simulink model "power_PVArray_PartialShading_Project"  (R2015a)
settings: Solver=ode23tb  SolverMode=SingleTasking  StartTime=0.0  StopTime=3  FixedStep=Ts_Power  RelTol=1e-4
PreLoadFcn:
  | Ts_Power=50e-6;
  | Slope_Vdc=1;
InitFcn:
  | Ts_Power=50e-6;
  | Tc=1e-5;%break algebraic loop time constant
  | BlockName=[gcs,'/4X4 PV Array/PV cells 1'];
  | ModuleName=get_param(BlockName,'ModuleName');
  | Voc1=str2num(get_param(BlockName,'Voc'));
  | Nser1=str2num(get_param(BlockName,'Nser'));
  | Slope_Vdc=Nser1*Voc1;
StopFcn:
  | if exist('I','var') && exist('V','var')
  |    figure(1)
  |    clf
  |    n=find(I>=0);
  |    n=n(end);
  |    Vglobal=V(1:n);
  |    Iglobal=I(1:n);
  | 
  | 
  |    Pglobal=Vglobal.*Iglobal;
  |    n=find(Pglobal==max(Pglobal));
  |    Pmax=Pglobal(n);
  |    Vmp=Vglobal(n);
  |    Imp=Iglobal(n);
  | 
  | 
  |    subplot(211)
  |    plot(Vglobal, Iglobal,Vmp,Imp,'or')
  |    ylabel('Current (A)')
  |    title(sprintf('Global I-V & P-V characteristics\n %s' ,ModuleName))
  | 
  | 
  |    subplot(212)
  |    plot(Vglobal, Pglobal,Vmp,Pmax,'or')
  |    ylabel('Power (W)')
  |    xlabel('Voltage (V)')
  | end
libraries: powerlib x20, re_lib x16, simulink x1
Description:
  | Copyright 2008-2015 The MathWorks, Inc.
settings Model: CovSFcnEnable=off  Creator=MathWorks  LastModifiedBy=Student
settings SolverCC: AlgebraicLoopSolver=LineSearch
settings DataIOCC: SignalLoggingSaveFormat=ModelDataLogs
settings OptimizationCC: ExpressionDepthLimit=2147483647
settings DebuggingCC: UnderspecifiedInitializationDetection=Classic  MergeDetectMultiDrivingBlocksExec=none  MaxConsecutiveZCsMsg=none  SolverPrmCheckMsg=warning  FcnCallInpInsideContextMsg=EnableAllAsWarning  StateNameClashWarn=warning
settings GRTTargetCC: CombineOutputUpdateFcns=off  GRTInterface=on

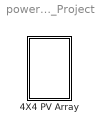
== system power_PVArray_PartialShading_Project ==
  4X4 PV Array : Subsystem  mask{Shade_A=900, Shade_B=600, Shade_C=300, Shade_D=100, No_Shade=1000}
      mask prompts: Shade_A "Shade - A"; Shade_B "Shade - B"; Shade_C "Shade - C"; Shade_D "Shade - D"

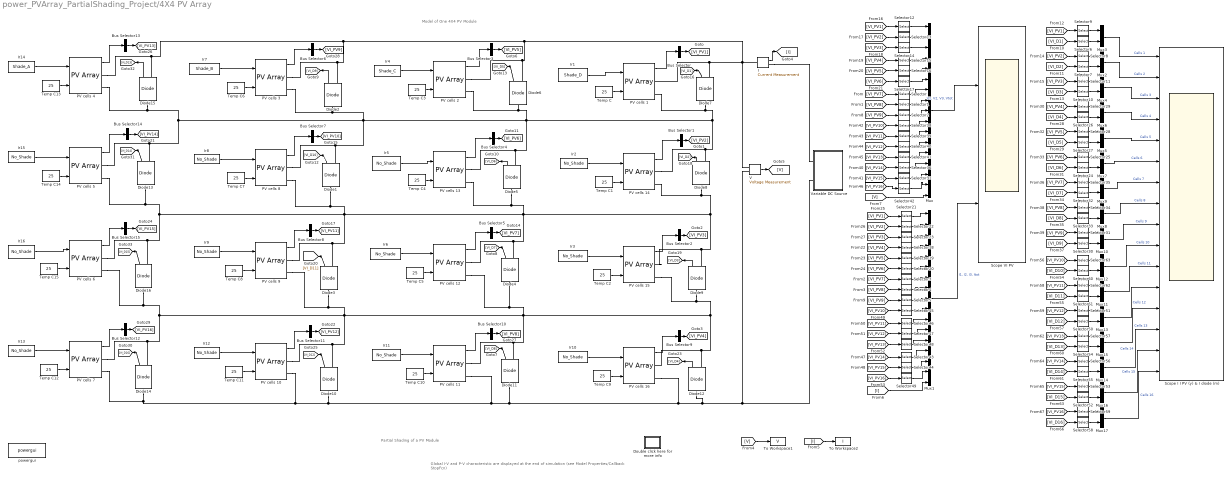
== system power_PVArray_PartialShading_Project/4X4 PV Array ==
  note: Model of One 4X4 PV Module
  note: Global I-V and P-V characteristic are displayed at the end of simulation
      | (see Model Properties/Callback StopFcn)
  note: Partial Shading of a PV Module
  Bus Selector{,1..15} (16 alike) : BusSelector  OutputSignals=V_PV,I_PV  OutputAsBus=on
  Diode{1..16} (16 alike) : powerlib/Power Electronics/Diode  Ron=0.001  Lon=0  Vf=0.7  IC=0  UseSnubber=off  Rs=1e5*inf  Cs=inf  Measurements=on
  Double click here for more info : Subsystem
      settings: OpenFcn=showdemo(bdroot(gcb))
      mask Display: disp('?')
  I : powerlib/Measurements/Current Measurement  PhasorSimulation=off  OutputType=Complex  PSBequivalent=0
  Ir1 : Constant  Value=Shade_D
  Ir{2..3,5..6,8..13,15..16} (12 alike) : Constant  Value=No_Shade
  Ir14 : Constant  Value=Shade_A
  Ir4 : Constant  Value=Shade_C
  Ir7 : Constant  Value=Shade_B
  Mux : Mux  Inputs=17
  Mux1 : Mux  Inputs=17
  Mux{2..17} (16 alike) : Mux  Inputs=2
  PV cells 1 : re_lib/Solar/PV Array  Npar=1  Nser=1  PlotType=array @ 25 deg.C & specified irradiances  S_vec="[ 1000  500  100 ]"  Temp_C_vec="[ 45 25  ]"  ModuleName=User-defined  PlotWhenSelected=off  Pm=2.2246  Ncell=1  Voc=0.7  Isc=4.74  Vm=17.64/36  Im=4.54  beta_Voc_pc=-0.33969  alpha_Isc_pc=0.063701  beta_Voc=-0.0023778  alpha_Isc=0.0030194  IL=4.8525  I0=7.8378e-11  nI=1.0965  Rsh=418.8028  Rs=0.030154  BAL=on  Tc=1  Tfilter=5e-5
      link override Diode Rsh/BAL/Transfer Fcn: Denominator="[Tc  1]"  AbsoluteTolerance=1e-3
  PV cells 10 : re_lib/Solar/PV Array  Npar=1  Nser=1  PlotType=array @ 25 deg.C & specified irradiances  S_vec="[ 1000  500  100 ]"  Temp_C_vec="[ 45 25  ]"  ModuleName=User-defined  PlotWhenSelected=off  Pm=2.2246  Ncell=1  Voc=0.7  Isc=4.74  Vm=17.64/36  Im=4.54  beta_Voc_pc=-0.33969  alpha_Isc_pc=0.063701  beta_Voc=-0.0023778  alpha_Isc=0.0030194  IL=4.8525  I0=7.8378e-11  nI=1.0965  Rsh=418.8028  Rs=0.030154  BAL=on  Tc=1  Tfilter=5e-5
      link override Diode Rsh/BAL/Transfer Fcn: Denominator="[Tc  1]"  AbsoluteTolerance=1e-3
  PV cells 11 : re_lib/Solar/PV Array  Npar=1  Nser=1  PlotType=array @ 25 deg.C & specified irradiances  S_vec="[ 1000  500  100 ]"  Temp_C_vec="[ 45 25  ]"  ModuleName=User-defined  PlotWhenSelected=off  Pm=2.2246  Ncell=1  Voc=0.7  Isc=4.74  Vm=17.64/36  Im=4.54  beta_Voc_pc=-0.33969  alpha_Isc_pc=0.063701  beta_Voc=-0.0023778  alpha_Isc=0.0030194  IL=4.8525  I0=7.8378e-11  nI=1.0965  Rsh=418.8028  Rs=0.030154  BAL=on  Tc=1  Tfilter=5e-5
      link override Diode Rsh/BAL/Transfer Fcn: Denominator="[Tc  1]"  AbsoluteTolerance=1e-3
  PV cells 12 : re_lib/Solar/PV Array  Npar=1  Nser=1  PlotType=array @ 25 deg.C & specified irradiances  S_vec="[ 1000  500  100 ]"  Temp_C_vec="[ 45 25  ]"  ModuleName=User-defined  PlotWhenSelected=off  Pm=2.2246  Ncell=1  Voc=0.7  Isc=4.74  Vm=17.64/36  Im=4.54  beta_Voc_pc=-0.33969  alpha_Isc_pc=0.063701  beta_Voc=-0.0023778  alpha_Isc=0.0030194  IL=4.8525  I0=7.8378e-11  nI=1.0965  Rsh=418.8028  Rs=0.030154  BAL=on  Tc=1  Tfilter=5e-5
      link override Diode Rsh/BAL/Transfer Fcn: Denominator="[Tc  1]"  AbsoluteTolerance=1e-3
  PV cells 13 : re_lib/Solar/PV Array  Npar=1  Nser=1  PlotType=array @ 25 deg.C & specified irradiances  S_vec="[ 1000  500  100 ]"  Temp_C_vec="[ 45 25  ]"  ModuleName=User-defined  PlotWhenSelected=off  Pm=2.2246  Ncell=1  Voc=0.7  Isc=4.74  Vm=17.64/36  Im=4.54  beta_Voc_pc=-0.33969  alpha_Isc_pc=0.063701  beta_Voc=-0.0023778  alpha_Isc=0.0030194  IL=4.8525  I0=7.8378e-11  nI=1.0965  Rsh=418.8028  Rs=0.030154  BAL=on  Tc=1  Tfilter=5e-5
      link override Diode Rsh/BAL/Transfer Fcn: Denominator="[Tc  1]"  AbsoluteTolerance=1e-3
  PV cells 14 : re_lib/Solar/PV Array  Npar=1  Nser=1  PlotType=array @ 25 deg.C & specified irradiances  S_vec="[ 1000  500  100 ]"  Temp_C_vec="[ 45 25  ]"  ModuleName=User-defined  PlotWhenSelected=off  Pm=2.2246  Ncell=1  Voc=0.7  Isc=4.74  Vm=17.64/36  Im=4.54  beta_Voc_pc=-0.33969  alpha_Isc_pc=0.063701  beta_Voc=-0.0023778  alpha_Isc=0.0030194  IL=4.8525  I0=7.8378e-11  nI=1.0965  Rsh=418.8028  Rs=0.030154  BAL=on  Tc=1  Tfilter=5e-5
      link override Diode Rsh/BAL/Transfer Fcn: Denominator="[Tc  1]"  AbsoluteTolerance=1e-3
  PV cells 15 : re_lib/Solar/PV Array  Npar=1  Nser=1  PlotType=array @ 25 deg.C & specified irradiances  S_vec="[ 1000  500  100 ]"  Temp_C_vec="[ 45 25  ]"  ModuleName=User-defined  PlotWhenSelected=off  Pm=2.2246  Ncell=1  Voc=0.7  Isc=4.74  Vm=17.64/36  Im=4.54  beta_Voc_pc=-0.33969  alpha_Isc_pc=0.063701  beta_Voc=-0.0023778  alpha_Isc=0.0030194  IL=4.8525  I0=7.8378e-11  nI=1.0965  Rsh=418.8028  Rs=0.030154  BAL=on  Tc=1  Tfilter=5e-5
      link override Diode Rsh/BAL/Transfer Fcn: Denominator="[Tc  1]"  AbsoluteTolerance=1e-3
  PV cells 16 : re_lib/Solar/PV Array  Npar=1  Nser=1  PlotType=array @ 25 deg.C & specified irradiances  S_vec="[ 1000  500  100 ]"  Temp_C_vec="[ 45 25  ]"  ModuleName=User-defined  PlotWhenSelected=off  Pm=2.2246  Ncell=1  Voc=0.7  Isc=4.74  Vm=17.64/36  Im=4.54  beta_Voc_pc=-0.33969  alpha_Isc_pc=0.063701  beta_Voc=-0.0023778  alpha_Isc=0.0030194  IL=4.8525  I0=7.8378e-11  nI=1.0965  Rsh=418.8028  Rs=0.030154  BAL=on  Tc=1  Tfilter=5e-5
      link override Diode Rsh/BAL/Transfer Fcn: Denominator="[Tc  1]"  AbsoluteTolerance=1e-3
  PV cells 2 : re_lib/Solar/PV Array  Npar=1  Nser=1  PlotType=array @ 25 deg.C & specified irradiances  S_vec="[ 1000  500  100 ]"  Temp_C_vec="[ 45 25  ]"  ModuleName=User-defined  PlotWhenSelected=off  Pm=2.2246  Ncell=1  Voc=0.7  Isc=4.74  Vm=17.64/36  Im=4.54  beta_Voc_pc=-0.33969  alpha_Isc_pc=0.063701  beta_Voc=-0.0023778  alpha_Isc=0.0030194  IL=4.8525  I0=7.8378e-11  nI=1.0965  Rsh=418.8028  Rs=0.030154  BAL=on  Tc=1  Tfilter=5e-5
      link override Diode Rsh/BAL/Transfer Fcn: Denominator="[Tc  1]"  AbsoluteTolerance=1e-3
  PV cells 3 : re_lib/Solar/PV Array  Npar=1  Nser=1  PlotType=array @ 25 deg.C & specified irradiances  S_vec="[ 1000  500  100 ]"  Temp_C_vec="[ 45 25  ]"  ModuleName=User-defined  PlotWhenSelected=off  Pm=2.2246  Ncell=1  Voc=0.7  Isc=4.74  Vm=17.64/36  Im=4.54  beta_Voc_pc=-0.33969  alpha_Isc_pc=0.063701  beta_Voc=-0.0023778  alpha_Isc=0.0030194  IL=4.8525  I0=7.8378e-11  nI=1.0965  Rsh=418.8028  Rs=0.030154  BAL=on  Tc=1  Tfilter=5e-5
      link override Diode Rsh/BAL/Transfer Fcn: Denominator="[Tc  1]"  AbsoluteTolerance=1e-3
  PV cells 4 : re_lib/Solar/PV Array  Npar=1  Nser=1  PlotType=array @ 25 deg.C & specified irradiances  S_vec="[ 1000  500  100 ]"  Temp_C_vec="[ 45 25  ]"  ModuleName=User-defined  PlotWhenSelected=off  Pm=2.2246  Ncell=1  Voc=0.7  Isc=4.74  Vm=17.64/36  Im=4.54  beta_Voc_pc=-0.33969  alpha_Isc_pc=0.063701  beta_Voc=-0.0023778  alpha_Isc=0.0030194  IL=4.8525  I0=7.8378e-11  nI=1.0965  Rsh=418.8028  Rs=0.030154  BAL=on  Tc=1  Tfilter=5e-5
      link override Diode Rsh/BAL/Transfer Fcn: Denominator="[Tc  1]"  AbsoluteTolerance=1e-3
  PV cells 5 : re_lib/Solar/PV Array  Npar=1  Nser=1  PlotType=array @ 25 deg.C & specified irradiances  S_vec="[ 1000  500  100 ]"  Temp_C_vec="[ 45 25  ]"  ModuleName=User-defined  PlotWhenSelected=off  Pm=2.2246  Ncell=1  Voc=0.7  Isc=4.74  Vm=17.64/36  Im=4.54  beta_Voc_pc=-0.33969  alpha_Isc_pc=0.063701  beta_Voc=-0.0023778  alpha_Isc=0.0030194  IL=4.8525  I0=7.8378e-11  nI=1.0965  Rsh=418.8028  Rs=0.030154  BAL=on  Tc=1  Tfilter=5e-5
      link override Diode Rsh/BAL/Transfer Fcn: Denominator="[Tc  1]"  AbsoluteTolerance=1e-3
  PV cells 6 : re_lib/Solar/PV Array  Npar=1  Nser=1  PlotType=array @ 25 deg.C & specified irradiances  S_vec="[ 1000  500  100 ]"  Temp_C_vec="[ 45 25  ]"  ModuleName=User-defined  PlotWhenSelected=off  Pm=2.2246  Ncell=1  Voc=0.7  Isc=4.74  Vm=17.64/36  Im=4.54  beta_Voc_pc=-0.33969  alpha_Isc_pc=0.063701  beta_Voc=-0.0023778  alpha_Isc=0.0030194  IL=4.8525  I0=7.8378e-11  nI=1.0965  Rsh=418.8028  Rs=0.030154  BAL=on  Tc=1  Tfilter=5e-5
      link override Diode Rsh/BAL/Transfer Fcn: Denominator="[Tc  1]"  AbsoluteTolerance=1e-3
  PV cells 7 : re_lib/Solar/PV Array  Npar=1  Nser=1  PlotType=array @ 25 deg.C & specified irradiances  S_vec="[ 1000  500  100 ]"  Temp_C_vec="[ 45 25  ]"  ModuleName=User-defined  PlotWhenSelected=off  Pm=2.2246  Ncell=1  Voc=0.7  Isc=4.74  Vm=17.64/36  Im=4.54  beta_Voc_pc=-0.33969  alpha_Isc_pc=0.063701  beta_Voc=-0.0023778  alpha_Isc=0.0030194  IL=4.8525  I0=7.8378e-11  nI=1.0965  Rsh=418.8028  Rs=0.030154  BAL=on  Tc=1  Tfilter=5e-5
      link override Diode Rsh/BAL/Transfer Fcn: Denominator="[Tc  1]"  AbsoluteTolerance=1e-3
  PV cells 8 : re_lib/Solar/PV Array  Npar=1  Nser=1  PlotType=array @ 25 deg.C & specified irradiances  S_vec="[ 1000  500  100 ]"  Temp_C_vec="[ 45 25  ]"  ModuleName=User-defined  PlotWhenSelected=off  Pm=2.2246  Ncell=1  Voc=0.7  Isc=4.74  Vm=17.64/36  Im=4.54  beta_Voc_pc=-0.33969  alpha_Isc_pc=0.063701  beta_Voc=-0.0023778  alpha_Isc=0.0030194  IL=4.8525  I0=7.8378e-11  nI=1.0965  Rsh=418.8028  Rs=0.030154  BAL=on  Tc=1  Tfilter=5e-5
      link override Diode Rsh/BAL/Transfer Fcn: Denominator="[Tc  1]"  AbsoluteTolerance=1e-3
  PV cells 9 : re_lib/Solar/PV Array  Npar=1  Nser=1  PlotType=array @ 25 deg.C & specified irradiances  S_vec="[ 1000  500  100 ]"  Temp_C_vec="[ 45 25  ]"  ModuleName=User-defined  PlotWhenSelected=off  Pm=2.2246  Ncell=1  Voc=0.7  Isc=4.74  Vm=17.64/36  Im=4.54  beta_Voc_pc=-0.33969  alpha_Isc_pc=0.063701  beta_Voc=-0.0023778  alpha_Isc=0.0030194  IL=4.8525  I0=7.8378e-11  nI=1.0965  Rsh=418.8028  Rs=0.030154  BAL=on  Tc=1  Tfilter=5e-5
      link override Diode Rsh/BAL/Transfer Fcn: Denominator="[Tc  1]"  AbsoluteTolerance=1e-3
  Scope I I PV (y) & I diode (m) : Scope  NumInputPorts=16
      settings: TimeRange=3  YMin=-2~-2~-2~-5~-5~-5~-5~-5~-5~-5~-5~-5~-5~-5~-5~-5  YMax=10~10~10~5~5~5~5~5~5~5~5~5~5~5~5~5  SaveName=VI1  SampleInput=on  SampleTime=5/1000
  Scope VI PV : Scope  NumInputPorts=2
      settings: TimeRange=3  YMin=-10~-2  YMax=40~10  SaveName=VI  SampleInput=on  SampleTime=5/1000
  Selector{,1..2,6..7,10,12..17,24,26..27,30,32..33,36..50,52,54..55,58,60..61} (39 alike) : Selector  InputPortWidth=2  Indices=[1]
  Selector{3..5,8..9,11,18..23,25,28..29,31,34..35,51,53,56..57,59,62..63} (25 alike) : Selector  InputPortWidth=2  Indices=[2]
  Temp C{,1..15} (16 alike) : Constant  Value=25
  To Workspace1 : ToWorkspace  VariableName=V  SampleTime=1e-3
  To Workspace2 : ToWorkspace  VariableName=I  SampleTime=1e-3
  V : powerlib/Measurements/Voltage Measurement  PhasorSimulation=off  OutputType=Complex  PSBequivalent=0
  Variable DC Source : Subsystem
  powergui : powerlib/powergui  Priority=1  SimulationMode=Continuous  SolverType=Tustin/Backward Euler (TBE)  SampleTime=Ts_Power*0 + 20e-6  frequency=60  SPID=off  DisableSnubberDevices=on  DisableRonSwitches=off  DisableVfSwitches=off  SwTol=0  DisplayEquations=off  Interpol=off  methode=off  Ts=0  FunctionMessages=off  echomessages=off  HookPort=off  EnableUseOfTLC=off  x0status=blocks  frequencyindice=0  Pbase=100e6  ErrMax=1e-4  Iterations=50  UnitsV=kV  UnitsW=MW  buscounter=0  RestoreLinks=warning  ResistiveCurrentMeasurement=off  Frange=[0:2:500]  Ylog=off  Xlog=on  ShowGrid=off  save=off  variable=ZData  structure=0  ZoomFFT=on  StartTime=0.0  cycles=1  DisplayStyle=1  fundamental=60  FreqAxis=off  MaxFrequency=1000  frequencyindicesteady=1  RmsSteady=1  display=off
  wires:
  Diode2/1 -> [VI_D9]
  Diode8/1 -> [VI_D2]
  Diode7/1 -> [VI_D1]
  Diode6/1 -> [VI_D5]
  Diode9/1 -> [VI_D3]
  PV cells 8/1 -> Bus Selector7/1
  Diode3/1 -> [VI_D11]
  Bus Selector8/1 -> [VI_PV11]
  Diode5/1 -> [VI_D6]
  Diode4/1 -> [VI_D7]
  PV cells 9/1 -> Bus Selector8/1
  Diode1/1 -> [VI_D10]
  Bus Selector7/1 -> [VI_PV10]
  Ir1/1 -> PV cells 1/1
  Ir4/1 -> PV cells 2/1
  Temp C1/1 -> PV cells 14/2
  Ir3/1 -> PV cells 15/1
  Ir6/1 -> PV cells 12/1
  Temp C/1 -> PV cells 1/2
  Bus Selector1/1 -> [VI_PV2]
  PV cells 14/1 -> Bus Selector1/1
  Bus Selector/1 -> [VI_PV1]
  Temp C3/1 -> PV cells 2/2
  PV cells 3/1 -> Bus Selector6/1
  Temp C7/1 -> PV cells 8/2
  PV cells 1/1 -> Bus Selector/1
  PV cells 15/1 -> Bus Selector2/1
  Temp C4/1 -> PV cells 13/2
  Ir2/1 -> PV cells 14/1
  Bus Selector5/1 -> [VI_PV7]
  Ir9/1 -> PV cells 9/1
  Ir7/1 -> PV cells 3/1
  Bus Selector2/1 -> [VI_PV3]
  Temp C5/1 -> PV cells 12/2
  I/1 -> [I]
  PV cells 2/1 -> Bus Selector3/1
  PV cells 13/1 -> Bus Selector4/1
  Ir5/1 -> PV cells 13/1
  V/1 -> [V]
  Temp C8/1 -> PV cells 9/2
  Ir8/1 -> PV cells 8/1
  Bus Selector3/1 -> [VI_PV5]
  PV cells 12/1 -> Bus Selector5/1
  Temp C2/1 -> PV cells 15/2
  Temp C6/1 -> PV cells 3/2
  Bus Selector6/1 -> [VI_PV9]
  Bus Selector4/1 -> [VI_PV6]
  Mux/1 -> Scope VI PV/1  "V1, V2, V3, Vtot"
  [V] -> Mux/17
  [VI_PV7] -> Selector/1
  [VI_PV8] -> Selector1/1
  [VI_PV9] -> Selector2/1
  Selector/1 -> Mux/7
  Selector1/1 -> Mux/8
  Selector2/1 -> Mux/9
  Mux1/1 -> Scope VI PV/2  "I1, I2, I3, Itot"
  [I] -> Mux1/17
  [VI_PV7] -> Selector3/1
  [VI_PV8] -> Selector4/1
  [VI_PV9] -> Selector5/1
  Selector3/1 -> Mux1/7
  Selector4/1 -> Mux1/8
  Selector5/1 -> Mux1/9
  [V] -> To Workspace1/1
  [I] -> To Workspace2/1
  [VI_PV1] -> Selector12/1
  [VI_PV2] -> Selector13/1
  [VI_PV3] -> Selector14/1
  Selector12/1 -> Mux/1
  Selector13/1 -> Mux/2
  Selector14/1 -> Mux/3
  [VI_PV4] -> Selector15/1
  [VI_PV5] -> Selector16/1
  [VI_PV6] -> Selector17/1
  Selector15/1 -> Mux/4
  Selector16/1 -> Mux/5
  Selector17/1 -> Mux/6
  [VI_PV4] -> Selector18/1
  [VI_PV5] -> Selector19/1
  [VI_PV6] -> Selector20/1
  Selector18/1 -> Mux1/4
  Selector19/1 -> Mux1/5
  Selector20/1 -> Mux1/6
  [VI_PV1] -> Selector21/1
  [VI_PV2] -> Selector22/1
  [VI_PV3] -> Selector23/1
  Selector21/1 -> Mux1/1
  Selector22/1 -> Mux1/2
  Selector23/1 -> Mux1/3
  [VI_PV1] -> Selector9/1
  Mux3/1 -> Scope I I PV (y) & I diode (m)/1  "Cells 1"
  Selector9/1 -> Mux3/1
  [VI_D1] -> Selector6/1
  Selector6/1 -> Mux3/2
  [VI_PV2] -> Selector8/1
  Mux2/1 -> Scope I I PV (y) & I diode (m)/2  "Cells 2"
  Selector8/1 -> Mux2/1
  [VI_D2] -> Selector7/1
  Selector7/1 -> Mux2/2
  [VI_PV3] -> Selector11/1
  Mux4/1 -> Scope I I PV (y) & I diode (m)/3  "Cells 3"
  Selector11/1 -> Mux4/1
  [VI_D3] -> Selector10/1
  Selector10/1 -> Mux4/2
  [VI_PV4] -> Selector29/1
  Mux6/1 -> Scope I I PV (y) & I diode (m)/4  "Cells 4"
  Selector29/1 -> Mux6/1
  [VI_D4] -> Selector26/1
  Selector26/1 -> Mux6/2
  [VI_PV5] -> Selector28/1
  Mux5/1 -> Scope I I PV (y) & I diode (m)/5  "Cells 5"
  Selector28/1 -> Mux5/1
  [VI_D5] -> Selector27/1
  Selector27/1 -> Mux5/2
  [VI_PV6] -> Selector25/1
  Mux7/1 -> Scope I I PV (y) & I diode (m)/6  "Cells 6"
  Selector25/1 -> Mux7/1
  [VI_D6] -> Selector24/1
  Selector24/1 -> Mux7/2
  [VI_PV7] -> Selector35/1
  Mux9/1 -> Scope I I PV (y) & I diode (m)/7  "Cells 7"
  Selector35/1 -> Mux9/1
  [VI_D7] -> Selector32/1
  Selector32/1 -> Mux9/2
  [VI_PV8] -> Selector34/1
  Mux8/1 -> Scope I I PV (y) & I diode (m)/8  "Cells 8"
  Selector34/1 -> Mux8/1
  [VI_D8] -> Selector33/1
  Selector33/1 -> Mux8/2
  [VI_PV9] -> Selector31/1
  Mux10/1 -> Scope I I PV (y) & I diode (m)/9  "Cells 9"
  Selector31/1 -> Mux10/1
  [VI_D9] -> Selector30/1
  Selector30/1 -> Mux10/2
  Diode12/1 -> [VI_D4]
  Diode10/1 -> [VI_D12]
  Bus Selector11/1 -> [VI_PV12]
  Diode11/1 -> [VI_D8]
  PV cells 10/1 -> Bus Selector11/1
  Ir10/1 -> PV cells 16/1
  Ir11/1 -> PV cells 11/1
  PV cells 16/1 -> Bus Selector9/1
  Bus Selector10/1 -> [VI_PV8]
  Ir12/1 -> PV cells 10/1
  Bus Selector9/1 -> [VI_PV4]
  Temp C10/1 -> PV cells 11/2
  Temp C11/1 -> PV cells 10/2
  PV cells 11/1 -> Bus Selector10/1
  Temp C9/1 -> PV cells 16/2
  Diode15/1 -> [VI_D13]
  PV cells 5/1 -> Bus Selector14/1
  Diode16/1 -> [VI_D15]
  Bus Selector15/1 -> [VI_PV15]
  PV cells 6/1 -> Bus Selector15/1
  Diode13/1 -> [VI_D14]
  Bus Selector14/1 -> [VI_PV14]
  PV cells 4/1 -> Bus Selector13/1
  Temp C14/1 -> PV cells 5/2
  Ir16/1 -> PV cells 6/1
  Ir14/1 -> PV cells 4/1
  Temp C15/1 -> PV cells 6/2
  Ir15/1 -> PV cells 5/1
  Temp C13/1 -> PV cells 4/2
  Bus Selector13/1 -> [VI_PV13]
  Diode14/1 -> [VI_D16]
  Bus Selector12/1 -> [VI_PV16]
  PV cells 7/1 -> Bus Selector12/1
  Ir13/1 -> PV cells 7/1
  Temp C12/1 -> PV cells 7/2
  [VI_PV14] -> Selector36/1
  [VI_PV15] -> Selector37/1
  [VI_PV16] -> Selector42/1
  Selector36/1 -> Mux/14
  Selector37/1 -> Mux/15
  Selector42/1 -> Mux/16
  [VI_PV10] -> Selector38/1
  Selector38/1 -> Mux/10
  [VI_PV11] -> Selector39/1
  [VI_PV12] -> Selector40/1
  [VI_PV13] -> Selector41/1
  Selector39/1 -> Mux/11
  Selector40/1 -> Mux/12
  Selector41/1 -> Mux/13
  [VI_PV14] -> Selector43/1
  [VI_PV15] -> Selector44/1
  [VI_PV16] -> Selector49/1
  Selector43/1 -> Mux1/14
  Selector44/1 -> Mux1/15
  Selector49/1 -> Mux1/16
  [VI_PV10] -> Selector45/1
  Selector45/1 -> Mux1/10
  [VI_PV11] -> Selector46/1
  [VI_PV12] -> Selector47/1
  [VI_PV13] -> Selector48/1
  Selector46/1 -> Mux1/11
  Selector47/1 -> Mux1/12
  Selector48/1 -> Mux1/13
  [VI_PV10] -> Selector63/1
  Mux12/1 -> Scope I I PV (y) & I diode (m)/10  "Cells 10"
  Selector63/1 -> Mux12/1
  [VI_D10] -> Selector60/1
  Selector60/1 -> Mux12/2
  [VI_PV11] -> Selector62/1
  Mux11/1 -> Scope I I PV (y) & I diode (m)/11  "Cells 11"
  Selector62/1 -> Mux11/1
  [VI_D11] -> Selector61/1
  Selector61/1 -> Mux11/2
  [VI_PV12] -> Selector51/1
  Mux13/1 -> Scope I I PV (y) & I diode (m)/12  "Cells 12"
  Selector51/1 -> Mux13/1
  [VI_D12] -> Selector50/1
  Selector50/1 -> Mux13/2
  [VI_PV13] -> Selector57/1
  Mux15/1 -> Scope I I PV (y) & I diode (m)/13  "Cells 13"
  Selector57/1 -> Mux15/1
  [VI_D13] -> Selector54/1
  Selector54/1 -> Mux15/2
  [VI_PV14] -> Selector56/1
  Mux14/1 -> Scope I I PV (y) & I diode (m)/14  "Cells 14"
  Selector56/1 -> Mux14/1
  [VI_D14] -> Selector55/1
  Selector55/1 -> Mux14/2
  [VI_PV15] -> Selector53/1
  Mux16/1 -> Scope I I PV (y) & I diode (m)/15  "Cells 15"
  Selector53/1 -> Mux16/1
  [VI_D15] -> Selector52/1
  Selector52/1 -> Mux16/2
  [VI_PV16] -> Selector59/1
  Mux17/1 -> Scope I I PV (y) & I diode (m)/16  "Cells 16"
  Selector59/1 -> Mux17/1
  [VI_D16] -> Selector58/1
  Selector58/1 -> Mux17/2
  connections:
  Diode13/LConn1 -- PV cells 5/RConn2 -- PV cells 12/RConn1 -- Diode4/RConn1 -- PV cells 13/RConn2 -- Diode5/LConn1 -- PV cells 14/RConn2 -- Diode8/LConn1 -- PV cells 15/RConn1 -- Diode9/RConn1 -- PV cells 9/RConn1 -- Diode3/RConn1 -- PV cells 8/RConn2 -- Diode1/LConn1 -- PV cells 6/RConn1 -- Diode16/RConn1
  Diode15/LConn1 -- PV cells 4/RConn2 -- PV cells 13/RConn1 -- Diode5/RConn1 -- PV cells 2/RConn2 -- Diode6/LConn1 -- Diode7/LConn1 -- PV cells 1/RConn2 -- PV cells 14/RConn1 -- Diode8/RConn1 -- PV cells 8/RConn1 -- Diode1/RConn1 -- PV cells 3/RConn2 -- Diode2/LConn1 -- PV cells 5/RConn1 -- Diode13/RConn1
  I/RConn1 -- Variable DC Source/LConn1
  PV cells 4/RConn1 -- Diode15/RConn1 -- Diode7/RConn1 -- PV cells 1/RConn1 -- V/LConn1 -- I/LConn1 -- PV cells 2/RConn1 -- Diode6/RConn1 -- PV cells 3/RConn1 -- Diode2/RConn1
  Diode16/LConn1 -- PV cells 6/RConn2 -- PV cells 15/RConn2 -- Diode9/LConn1 -- PV cells 16/RConn1 -- Diode12/RConn1 -- PV cells 12/RConn2 -- Diode4/LConn1 -- PV cells 11/RConn1 -- Diode11/RConn1 -- PV cells 10/RConn1 -- Diode10/RConn1 -- PV cells 9/RConn2 -- Diode3/LConn1 -- PV cells 7/RConn1 -- Diode14/RConn1
  PV cells 7/RConn2 -- Diode14/LConn1 -- PV cells 10/RConn2 -- PV cells 11/RConn2 -- PV cells 16/RConn2 -- Diode12/LConn1 -- Variable DC Source/LConn2 -- V/LConn2 -- Diode11/LConn1 -- Diode10/LConn1

== system power_PVArray_PartialShading_Project/4X4 PV Array/Double click here for more info ==

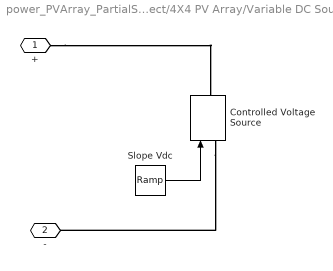
== system power_PVArray_PartialShading_Project/4X4 PV Array/Variable DC Source ==
  Controlled Voltage Source : powerlib/Electrical Sources/Controlled Voltage Source  Initialize=on  Source_Type=AC  Amplitude=0  Phase=0  Frequency=0  Measurements=None
  Slope Vdc : simulink/Sources/Ramp  slope=Slope_Vdc  start=0  X0=0
  + : PMIOPort  Port=1  Side=Left
  - : PMIOPort  Port=2  Side=Left
  wires:
  Slope Vdc/1 -> Controlled Voltage Source/1
  connections:
  Controlled Voltage Source/LConn1 -- -/RConn1
  +/RConn1 -- Controlled Voltage Source/RConn1
